simulink model "base98"  (Simulink 3.00)
settings: Solver=ode45  StartTime=0.0  StopTime=999999  MaxStep=10  RelTol=1e-3  AbsTol=1e-3
undefined symbols (not defined in the file or in its folder): df2, offset, ssfunpsd
settings Model: SaveTime=off  SaveOutput=off

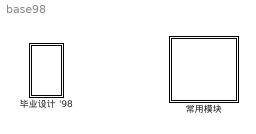
== system base98 ==
  毕业设计 '98 : Subsystem
  常用模块 : Subsystem
      settings: OpenFcn=axzblock
      mask Display: disp('模块库')

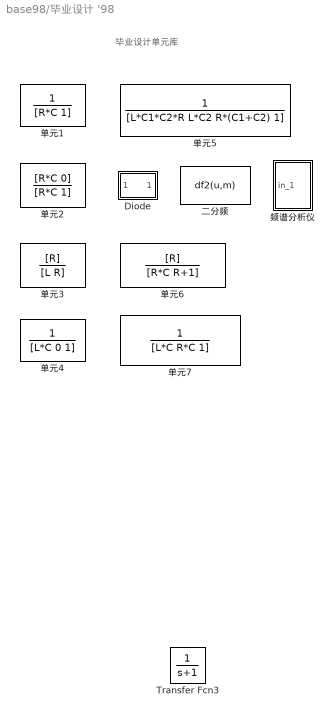
== system base98/毕业设计 '98 ==
  note: 毕业设计单元库
  Diode : Subsystem
      mask Type: 二极管
      mask Description: 二极管
      mask Display: plot([0 2 2 2],[0 0 2 -2],[2 4],[2 0],[2 4],[-2 0],[4 4 4 6],[-2 2 0 0]);
  Transfer Fcn3 : TransferFcn  Numerator=[1]  Denominator=[1 1]
  单元1 : TransferFcn  Numerator=[1]  Denominator=[R*C 1]  mask(积分){@1=1, @2=1}
      mask prompts: @1 "电容量（法）："; @2 "电阻值（欧姆）："
      mask help: 积分
      mask init:
      | C=@1;R=@2;
      mask Display: plot([0 2 2 2],[2 2 1.5 2.5],[2 6],[2.5 2.5],[2 6],[1.5 1.5],[6 6],[2.5 1.5],[6 11],[2 2],[8 8 6 10],[2 0 0 0],[6 10],[-1 -1],[8 8 7 9],[-1 -3 -3 -3]);
  单元2 : TransferFcn  Numerator=[R*C 0]  Denominator=[R*C 1]  mask(微分){@1=1, @2=1}
      mask prompts: @1 "电容量（法）："; @2 "电阻值（欧姆）："
      mask help: 微分
      mask init:
      | C=@1;R=@2;
      mask Display: plot([0 2 2 2],[2 2 0 4],[3 3 3 8],[0 4 2 2],[6 6 5.5 6.5],[2 0 0 0],[5.5 5.5],[0 -4],[6.5 6.5],[0 -4],[5.5 6.5 6 6],[-4 -4 -4 -5.5],[5.5 6.5],[-5.5 -5.5]);
  单元3 : TransferFcn  Numerator=[R]  Denominator=[L R]  mask(单元3){@1=1, @2=1}
      mask prompts: @1 "电感量（亨）："; @2 "电阻值（欧）："
      mask help: 单元3
      mask init:
      | L=@1;R=@2;
      mask Display: plot([0 1],[1 1],[1:1/7:2],[1 1.5 1.707 1.866 1.866 1.707 1.5 1],[2:1/7:3],[1 1.5 1.707 1.866 1.866 1.707 1.5 1],[3:1/7:4],[1 1.5 1.707 1.866 1.866 1.707 1.5 1],[4:1/7:5],[1 1.5 1.707 1.866 1.866 1.707 1.5 1],[5 8],[1 1],[6.5 6.5 6 7],[1 0 0 0],[6 6],[0 -4],[7 7],[0 -4],[6 7 6.5 6.5],[-4 -4 -4 -5.5],[6 7],[-5.5 -5.5])
  单元4 : TransferFcn  Numerator=[1]  Denominator=[L*C 0 1]  mask(单元4){@1=1, @2=1}
      mask prompts: @1 "电感量（亨）："; @2 "电容量（法）："
      mask help: 单元4
      mask init:
      | L=@1;C=@2;
      mask Display: plot([0 1],[1 1],[1:1/7:2],[1 1.5 1.707 1.866 1.866 1.707 1.5 1],[2:1/7:3],[1 1.5 1.707 1.866 1.866 1.707 1.5 1],[3:1/7:4],[1 1.5 1.707 1.866 1.866 1.707 1.5 1],[4:1/7:5],[1 1.5 1.707 1.866 1.866 1.707 1.5 1],[5 11],[1 1],[8 8 6 10],[1 -1 -1 -1],[6 10],[-2 -2],[8 8 7 9],[-2 -4 -4 -4]);
  单元5 : TransferFcn  Numerator=[1]  Denominator=[L*C1*C2*R L*C2 R*(C1+C2) 1]  mask(单元5){@1=1, @2=1, @3=1, @4=1}
      mask prompts: @1 "电阻R（欧）："; @2 "电容C1（法）："; @3 "电感L（亨）："; @4 "电容C2（法）："
      mask help: 单元5
      mask init:
      | R=@1;C1=@2;L=@3;C2=@4;
      mask Display: plot([0 2 2 2],[2 2 1.5 2.5],[2 6],[2.5 2.5],[2 6],[1.5 1.5],[6 6],[2.5 1.5],[6 11],[2 2],[8 8 6 10],[2 0 0 0],[6 10],[-1 -1],[8 8 7 9],[-1 -3 -3 -3],[11:1/7:12],[2 2.5 2.707 2.866 2.866 2.707 2.5 2],[12:1/7:13],[2 2.5 2.707 2.866 2.866 2.707 2.5 2],[13:1/7:14],[2 2.5 2.707 2.866 2.866 2.707 2.5 2],[14:1/7:15],[2 2.5 2.707 2.866 2.866 2.707 2.5 2],[15 21],[2 2],[18 18 16 20],[2 0 0 0],[16 20],[-1 -1],[18 18 17 19],[-1 -3 -3 -3]);disp('R     C1     L      C2')
  单元6 : TransferFcn  Numerator=[R]  Denominator=[R*C R+1]  mask(单元6){@1=1, @2=1}
      mask prompts: @1 "电阻值（欧）："; @2 "电容值（法）："
      mask help: 单元6
      mask init:
      | R=@1;C=@2;
      mask Display: plot([0 15],[2 2],[8 8 6 10],[2 0 0 0],[6 10],[-1 -1],[8 8 7 9],[-1 -4 -4 -4],[12.5 12.5 12 13],[2 1 1 1],[12 12],[1 -3],[13 13],[1 -3],[12 13 12.5 12.5],[-3 -3 -3 -4],[12 13],[-4 -4]);
  单元7 : TransferFcn  Numerator=[1]  Denominator=[L*C R*C 1]  mask( 单元7){@1=1, @2=1, @3=1}
      mask prompts: @1 "电阻值（欧）："; @2 "电感值（亨）："; @3 "电容值（法）："
      mask help: 单元7
      mask init:
      | R=@1;L=@2;C=@3;
      mask Display: plot([3 5 5 5],[2 2 1.5 2.5],[5 9],[2.5 2.5],[5 9],[1.5 1.5],[9 9],[2.5 1.5],[9 11],[2 2],[11:1/7:12],[2 2.5 2.707 2.866 2.866 2.707 2.5 2],[12:1/7:13],[2 2.5 2.707 2.866 2.866 2.707 2.5 2],[13:1/7:14],[2 2.5 2.707 2.866 2.866 2.707 2.5 2],[14:1/7:15],[2 2.5 2.707 2.866 2.866 2.707 2.5 2],[15 21],[2 2],[18 18 16 20],[2 0 0 0],[16 20],[-1 -1],[18 18 17 19],[-1 -3 -3 -3]);
  二分频 : MATLABFcn  MATLABFcn=df2(u,m)  OutputWidth=-1  OutputSignalType=auto  mask(分频器){@1=100}
      mask prompts: @1 "判决区间："
      mask help: 二分频器
      mask init:
      | m=@1;
      mask Display: disp('Frequency\n—————\n2')
  频谱分析仪 : Subsystem  LoadFcn=ssfunpsd([],[],[],'LoadBlock')  StartFcn=ssfunpsd([],[],[],'Start')  mask(频谱分析仪){@1=1024, @2=1024, @3=64, @4=0.01}
      mask prompts: @1 "缓冲区长度："; @2 "进行 FFT 运算的点数："; @3 "在多少点后画图："; @4 "采样周期："
      mask help: 频谱分析仪（利用图形窗口显示实时结果）
      mask init:
      | npts=@1; fftpts=@2; HowOften=@3; ts=@4(1); if length(@4) > 1, offset = @4(2), else, offset = 0; end
      settings: CopyFcn=ssfunpsd([],[],[],'CopyBlock')  DeleteFcn=ssfunpsd([],[],[],'DeleteBlock')  NameChangeFcn=ssfunpsd([],[],[],'NameChange')
      mask Help: 当把该模块连接到一个系统的输出时，将以图形窗口的方式显示出信号的频谱图。
      mask Display: plot(0,0,100,100,[14,91,91,14,14],[86,86,40,40,86],[85,82,80,79,75,67,63,60,57,53,41,36,33,27,24],[49,50,53,50,49,51,54,66,54,50,50,52,81,51,49])

== system base98/常用模块 ==

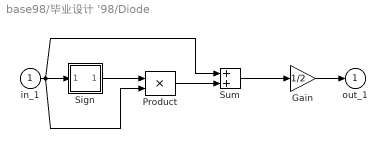
== system base98/毕业设计 '98/Diode ==
  in_1 : Inport  Port=1  PortWidth=-1  SampleTime=-1  DataType=auto
      settings: SignalType=auto
  Gain : Gain  Gain=1/2  SaturateOnIntegerOverflow=on
  Product : Product  Inputs=2  SaturateOnIntegerOverflow=on
  Sign : Subsystem
      mask Type: Sign
      mask Description: y = sign(x)
      mask Help: Sign Function:\n\t\t\ty = 1 if x > 0\n\t\t\ty = 0 if x = 0\n\t\t\ty = -1 if x < 0
      mask Display: plot(-50,-50,50,50,[-50,50],[0,0],[0,0],[-50,50],[-40,0],[-30,-30],[0,40],[30,30])
  Sum : Sum  Inputs=++  SaturateOnIntegerOverflow=on
  out_1 : Outport  Port=1
  wires:
  Sum/1 -> Gain/1
  Product/1 -> Sum/2
  in_1/1 -> Sum/1, Product/2, Sign/1(in_1)
  Sign/1(out_1) -> Product/1
  Gain/1 -> out_1/1

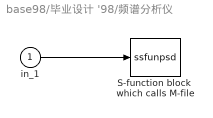
== system base98/毕业设计 '98/频谱分析仪 ==
  in_1 : Inport  Port=1  PortWidth=-1  SampleTime=-1  DataType=auto
      settings: SignalType=auto
  S-function block  which calls M-file : S-Function  FunctionName=ssfunpsd  Parameters=fftpts,npts,HowOften,offset,ts,0  PortCounts=[]  SFunctionModules=''
  wires:
  in_1/1 -> S-function block  which calls M-file/1

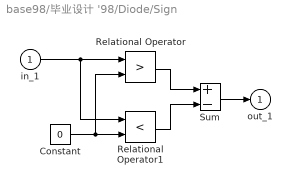
== system base98/毕业设计 '98/Diode/Sign ==
  in_1 : Inport  Port=1  PortWidth=-1  SampleTime=-1  DataType=auto
      settings: SignalType=auto
  Constant : Constant  Value=0
  Relational Operator : RelationalOperator  Operator=>
  Relational Operator1 : RelationalOperator  Operator=<
  Sum : Sum  Inputs=+-  SaturateOnIntegerOverflow=on
  out_1 : Outport  Port=1
  wires:
  in_1/1 -> Relational Operator/1, Relational Operator1/1
  Constant/1 -> Relational Operator1/2, Relational Operator/2
  Relational Operator1/1 -> Sum/2
  Relational Operator/1 -> Sum/1
  Sum/1 -> out_1/1
